simulink model "gyrocopy"  (R2022a)
settings: Solver=VariableStepAuto  StartTime=0.0  StopTime=10.0  RelTol=1e-3
settings Model: Creator=tobia  LastModifiedBy=tobia

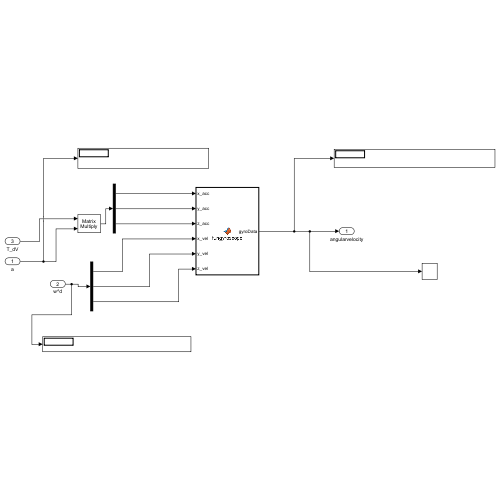
[thumbnail: Simulink's stored preview of the top-level diagram]
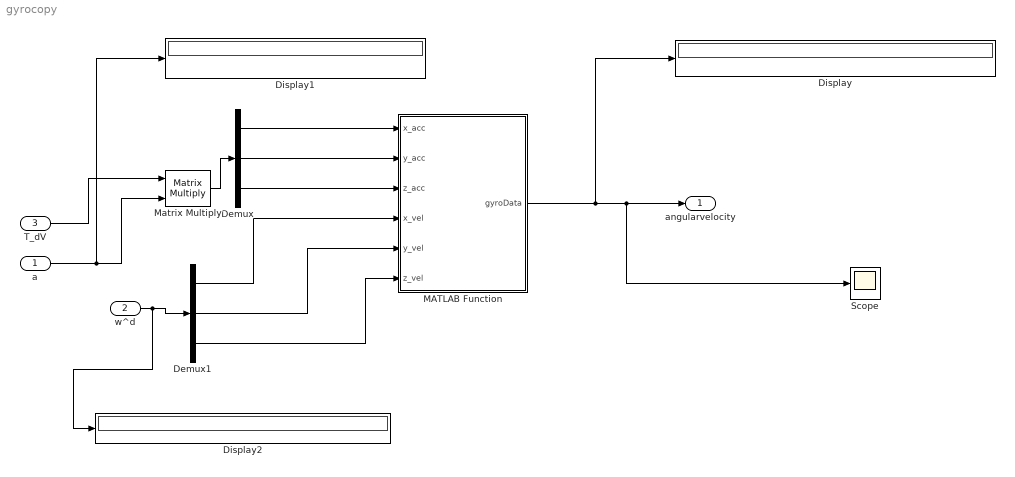
== system gyrocopy ==
  a : Inport
  w^d : Inport  Port=2
  T_dV : Inport  Port=3
  Demux : Demux  Outputs=3
  Demux1 : Demux  Outputs=3
  Display : Display
  Display1 : Display
  Display2 : Display
  MATLAB Function : MATLAB Function  TreatAsAtomicUnit=on
  Matrix Multiply : Product  Multiplication=Matrix(*)
  Scope : Scope
  angularvelocity : Outport
  wires:
  Demux/1 -> MATLAB Function/1(x_acc)
  Demux/2 -> MATLAB Function/2(y_acc)
  Demux/3 -> MATLAB Function/3(z_acc)
  MATLAB Function/1(gyroData) -> Display/1, Scope/1, angularvelocity/1
  Demux1/3 -> MATLAB Function/6(z_vel)
  Demux1/2 -> MATLAB Function/5(y_vel)
  Demux1/1 -> MATLAB Function/4(x_vel)
  w^d/1 -> Display2/1, Demux1/1
  Matrix Multiply/1 -> Demux/1
  a/1 -> Display1/1, Matrix Multiply/2
  T_dV/1 -> Matrix Multiply/1

== matlab function gyrocopy/MATLAB Function ==
  settings: updateMethod=DISCRETE
  data: x_acc input; gyroData output; y_acc input; z_acc input; x_vel input; y_vel input; z_vel input
function gyroData  = fungyroscope(x_acc, y_acc, z_acc, x_vel, y_vel, z_vel)
   
    % Create gyroscope sensor object
    params = gyroparams;         
    
    acc = [x_acc, y_acc, z_acc];
    angvel = [x_vel, y_vel, z_vel];

    % Parameters for simulated signal
    N = 1;       % Number of samples
    Fs = 100;       % Sampling rate
    Fc = 0.25;      % Sinusoidal frequency
    
    % Create arrays
    t = (0:(1/Fs):((N-1)/Fs)).';
    acc = acc;          % Input accelerations
    angvel = angvel;
    %angvel(:,1) = 8*sin(2*pi*Fc*t);
    
    % Generate gyroscopic data
    imu = imuSensor('SampleRate', Fs, 'Gyroscope', params);
    %imu.Gyroscope.MeasurementRange = 6.5;   % Maximum angular velocity gyroscope can measure
    imu.Gyroscope.Resolution = 1/Fs;           % Step size of digital measurements
    
    % Biases
    
    imu.Gyroscope.BiasInstability = 0.12 * 3.14159 / 180;       % rad/hr
    imu.Gyroscope.NoiseDensity = 0.15 * 3.14159 / 180;          % rad/s
    imu.Gyroscope.RandomWalk = 0.017 * 3.14159 / 180;           % rad/sqrt(hr)
    imu.Gyroscope.TemperatureBias = 0.25 * 3.14159 / 180;       % rad/s
    %imu.Gyroscope.AccelerationBias = 0.3;
    
    % Define real accelerations
    %acc(:,1) = 1;
    [~, gyroData] = imu(acc, angvel);

end
